simulink model "ob_ob_re"  (R2016b)
settings: Solver=ode4  StartTime=0.0  StopTime=15  FixedStep=0.01  RelTol=1e-3
values from neighbouring files (symbols this model uses):
  A = [2  -4  -1; 4  -2  -1; -4  0  -1]    [matlab.mat]    (also in obserwator_stanu.m = [2 -4 -1)
  Aa = 2    [matlab.mat]    (also in obserwator_stanu.m = Ac(1,1))
  Aab = [-4 -1]    [matlab.mat]    (also in obserwator_stanu.m = Ac(1,2:3))
  Ab = [-2  -1; -7.5  -3]    [matlab.mat]    (also in obserwator_stanu.m = Ac(2:3,2:3))
  Aba = [4 4]    [matlab.mat]    (also in obserwator_stanu.m = Ac(2:3,1))
  B = [0 0 -2]    [matlab.mat]    (also in obserwator_stanu.m = [0;0;-2])
  Ba = 0    [matlab.mat]    (also in obserwator_stanu.m = B(1,1))
  Bb = [0 -2]    [matlab.mat]    (also in obserwator_stanu.m = B(2:3,1))
  C = [1 0 0]    [matlab.mat]    (also in obserwator_stanu.m)
  D = 0    [matlab.mat]    (also in obserwator_stanu.m = [0])
  Hb = [-0.78 4.12]    [matlab.mat]    (also in obserwator_stanu.m = L_new')
  Ka = 4    [matlab.mat]    (also in obserwator_stanu.m = K(1,1))
  Kb = [-3.75 -1]    [matlab.mat]    (also in obserwator_stanu.m = K(1,2:3))
  Ki = 205    [matlab.mat]    (also in obserwator_stanu.m = K1(1,4))
  N = -3.25    [matlab.mat]    (also in obserwator_stanu.m = K*Nx+Nu)
undefined symbols (not defined in the file or in its folder): sigbuilder_block
settings Model: Creator=lenovo  LastModifiedBy=lenovo

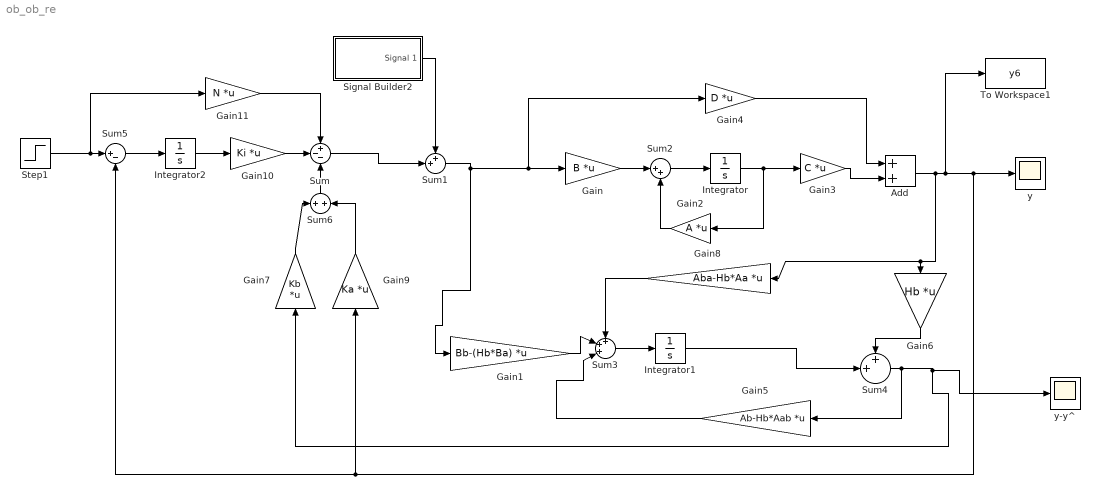
== system ob_ob_re ==
  Add : Sum
  Gain : Gain  Gain=B  Multiplication=Matrix(K*u)
  Gain1 : Gain  Gain=Bb-(Hb*Ba)  Multiplication=Matrix(K*u)
  Gain10 : Gain  Gain=Ki  Multiplication=Matrix(K*u)
  Gain11 : Gain  Gain=N  Multiplication=Matrix(K*u)
  Gain2 : Gain  Gain=A  Multiplication=Matrix(K*u)
  Gain3 : Gain  Gain=C  Multiplication=Matrix(K*u)
  Gain4 : Gain  Gain=D  Multiplication=Matrix(K*u)
  Gain5 : Gain  Gain=Ab-Hb*Aab  Multiplication=Matrix(K*u)
  Gain6 : Gain  Gain=Hb  Multiplication=Matrix(K*u)
  Gain7 : Gain  Gain=Kb  Multiplication=Matrix(K*u)
  Gain8 : Gain  Gain=Aba-Hb*Aa  Multiplication=Matrix(K*u)
  Gain9 : Gain  Gain=Ka  Multiplication=Matrix(K*u)
  Integrator : Integrator
  Integrator1 : Integrator
  Integrator2 : Integrator
  Signal Builder2 : Subsystem  Tag=STV Subsys  LoadFcn=sigbuilder_block('load');  StartFcn=sigbuilder_block('start');  StopFcn=sigbuilder_block('stop');  ClipboardFcn=sigbuilder_block('clipboard');  mask(Sigbuilder block){tuvar=[0:10]}
      mask help: Simulink:masks:SigbuilderBlock_MD
      mask init:
      | if ~strcmp(get_param(bdroot(gcbh),'SimulationStatus'),'stopped') tuvar = sigbuilder_block('maskInit'); end
      settings: CopyFcn=sigbuilder_block('copy');  DeleteFcn=sigbuilder_block('delete');  ModelCloseFcn=sigbuilder_block('modelClose');  PreSaveFcn=sigbuilder_block('preSave');  PauseFcn=sigbuilder_block('pause');  ContinueFcn=sigbuilder_block('continue');  NameChangeFcn=sigbuilder_block('namechange');  OpenFcn=sigbuilder_block('open',[437.25 153.75 550.5 359.25 ]);  CloseFcn=sigbuilder_block('close');
      mask Display: plot(0, 0, 100, 100,[2, 2, 32, 32, 2], [68, 8, 8, 68, 68],[32, 2], [38, 38], [32, 19, 2],[53, 60, 44], [32, 17, 17, 2],[16, 16, 31, 31]);txt = getActiveGroup(gcbh);text(2, 100, txt,'verticalAlignment', 'top');
  Step1 : Step  Time=0  SampleTime=0
  Sum : Sum  Inputs=+--
  Sum1 : Sum  Inputs=++|
  Sum2 : Sum  Inputs=|++
  Sum3 : Sum  Inputs=+++|
  Sum4 : Sum  Inputs=++|
  Sum5 : Sum  Inputs=|+-
  Sum6 : Sum  Inputs=+|+
  To Workspace1 : ToWorkspace  VariableName=y6  SaveFormat=Timeseries  SampleTime=-1
  y : Scope
  y-y^ : Scope
  wires:
  Gain2/1 -> Sum2/2
  Gain/1 -> Sum2/1
  Sum2/1 -> Integrator/1
  Integrator/1 -> Gain2/1, Gain3/1
  Gain3/1 -> Add/2
  Gain4/1 -> Add/1
  Sum3/1 -> Integrator1/1
  Gain1/1 -> Sum3/2
  Gain5/1 -> Sum3/3
  Gain8/1 -> Sum3/1
  Sum/1 -> Sum1/2
  Step1/1 -> Gain11/1, Sum5/1
  Sum5/1 -> Integrator2/1
  Integrator2/1 -> Gain10/1
  Gain10/1 -> Sum/2
  Gain11/1 -> Sum/1
  Sum1/1 -> Gain4/1, Gain/1, Gain1/1
  Add/1 -> Gain6/1, Gain8/1, To Workspace1/1, Gain9/1, Sum5/2, y/1
  Sum4/1 -> Gain5/1, y-y^/1, Gain7/1
  Integrator1/1 -> Sum4/2
  Gain6/1 -> Sum4/1
  Sum6/1 -> Sum/3
  Gain7/1 -> Sum6/1
  Gain9/1 -> Sum6/2
  Signal Builder2/1(Signal 1) -> Sum1/1

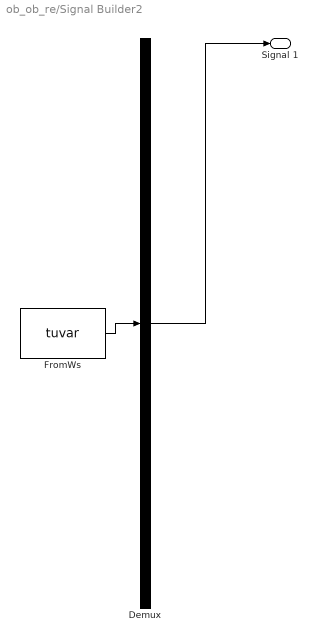
== system ob_ob_re/Signal Builder2 ==
  Demux : Demux  Tag=STV Demux  Outputs=1
  FromWs : FromWorkspace  Tag=STV FromWs  VariableName=tuvar  SampleTime=0
      SigBuilderData=|
      | common.afterFinalStr = 'Extrapolate'
      | common.sampleTime = 0
      | dataSet.timeRange = [0 10]
      | dataSet.name = 'Group 1'
      | sbobj.Groups.Name = 'Group 1'
      | sbobj.Groups.Signals.Name = 'Signal 1'
      | sbobj.Groups.Signals.XData = [0 7.22 7.22 7.46 7.46 10]
      | sbobj.Groups.Signals.YData = [0 0 1.005 1.005 0 0]
  Signal 1 : Outport  Tag=STV Outport
  wires:
  Demux/1 -> Signal 1/1
  FromWs/1 -> Demux/1
